simulink model "ACC_ensemble_training"  (R2022a)
settings: Solver=FixedStepAuto  StartTime=0.0  StopTime=T  FixedStep=Ts  RelTol=1e-3
InitFcn:
  | a_lead_seed = randi(10000);
StartFcn:
  | a_lead_seed = randi(10000);
undefined symbols (not defined in the file): actionUB, amax_ego, amax_lead, amin_ego, amin_lead, change_freq, D_default, ensembleRewardWeights, isEnsembleTerminate, isTerminate, MPC_ST, numController, numRL, rewardToIndex, rewardUB1, rewardUB2, rewardWeights, t_gap, tranTable, Ts, v0_ego, v0_lead, v_set, x0_ego, x0_lead
libraries: simulink x10, rllib x10, mpcadaslib x2
settings Model: Creator=The MathWorks, Inc.  LastModifiedBy=momentumlab
settings SolverCC: AlgebraicLoopSolver=TrustRegion
settings DataIOCC: ReturnWorkspaceOutputs=off
settings DebuggingCC: UnconnectedInputMsg=warning  UnconnectedOutputMsg=warning  UnconnectedLineMsg=warning  SFMachineParentedDataDiag=warning  ArithmeticOperatorsInVariantConditions=warning
settings SFSimCC: SimUseLocalCustomCode=off  CustomCodeUndefinedFunction=UseInterfaceOnly
settings RTWCC: RTWUseLocalCustomCode=off  DLArmComputeVersion=19.05
settings CodeAppCC: StateflowObjectComments=on

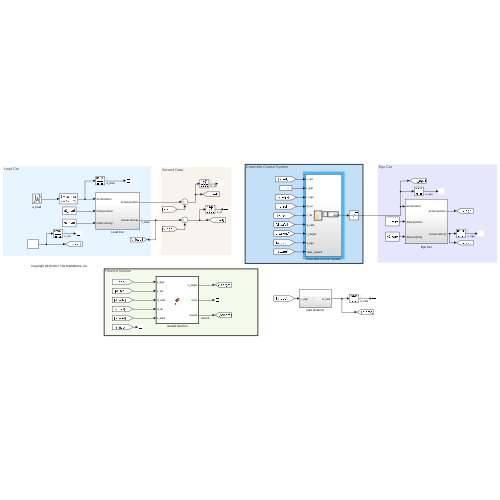
[thumbnail: Simulink's stored preview of the top-level diagram]
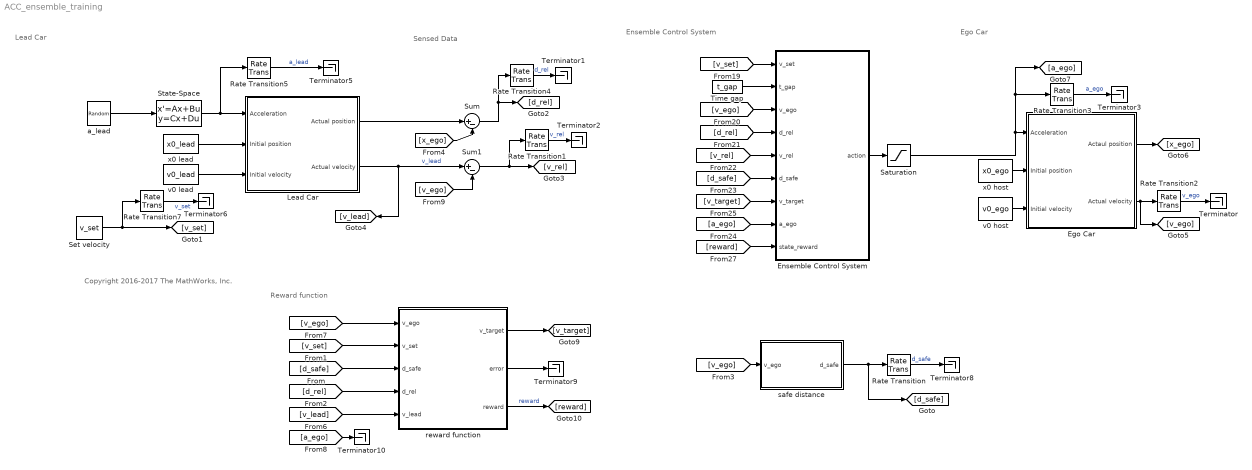
== system ACC_ensemble_training ==
  note: Ensemble Control System
  note: Sensed Data
  note: Lead Car
  note: Ego Car
  note: Copyright 2016-2017 The MathWorks, Inc.
  note: Reward function
  Ego Car : Subsystem
  Ensemble Control System : Subsystem
  Lead Car : Subsystem
  Rate Transition{,1..5,7} (7 alike) : RateTransition  OutPortSampleTime=Ts_data
  Saturation : Saturate  UpperLimit=amax_ego  LowerLimit=amin_ego
  Set velocity : Constant  Value=v_set  SampleTime=Ts
  State-Space : StateSpace  A=-10  B=10  D=0  InitialCondition=0
  Sum : Sum  Inputs=|+-
  Sum1 : Sum  Inputs=|+-
  Terminator{,1..3,5..6,8..10} (9 alike) : Terminator
  Time gap : Constant  Value=t_gap  SampleTime=Ts
  a_lead : UniformRandomNumber  Minimum=amin_lead  Maximum=amax_lead  Seed=a_lead_seed  SampleTime=change_freq  VectorParams1D=off
  reward function : MATLAB Function  TreatAsAtomicUnit=on
  safe distance : Subsystem
  v0 host : Constant  Value=v0_ego  SampleTime=Ts
  v0 lead : Constant  Value=v0_lead  SampleTime=Ts
  x0 host : Constant  Value=x0_ego  SampleTime=Ts
  x0 lead : Constant  Value=x0_lead  SampleTime=Ts
  wires:
  x0 lead/1 -> Lead Car/2(Initial position)
  v0 lead/1 -> Lead Car/3(Initial velocity)
  x0 host/1 -> Ego Car/2(Initial position)
  Ego Car/2(Actual velocity) -> [v_ego], Rate Transition2/1
  v0 host/1 -> Ego Car/3(Initial velocity)
  Set velocity/1 -> Rate Transition7/1, [v_set]
  Saturation/1 -> Ego Car/1(Acceleration), [a_ego], Rate Transition3/1
  Lead Car/1(Actual position) -> Sum/1
  Sum1/1 -> [v_rel], Rate Transition1/1
  State-Space/1 -> Rate Transition5/1, Lead Car/1(Acceleration)
  Lead Car/2(Actual velocity) -> Sum1/1, [v_lead]  "v_lead"
  Sum/1 -> [d_rel], Rate Transition4/1
  a_lead/1 -> State-Space/1
  safe distance/1(d_safe) -> [d_safe], Rate Transition/1
  Rate Transition/1 -> Terminator8/1  "d_safe"
  Rate Transition2/1 -> Terminator/1  "v_ego"
  Rate Transition3/1 -> Terminator3/1  "a_ego"
  Rate Transition5/1 -> Terminator5/1  "a_lead"
  [v_ego] -> safe distance/1(v_ego)
  Ego Car/1(Actaul position) -> [x_ego]
  Rate Transition4/1 -> Terminator1/1  "d_rel"
  Rate Transition1/1 -> Terminator2/1  "v_rel"
  [x_ego] -> Sum/2
  [v_ego] -> Sum1/2
  Rate Transition7/1 -> Terminator6/1  "v_set"
  Ensemble Control System/1(action) -> Saturation/1
  [v_set] -> Ensemble Control System/1(v_set)
  Time gap/1 -> Ensemble Control System/2(t_gap)
  [v_ego] -> Ensemble Control System/3(v_ego)
  [d_rel] -> Ensemble Control System/4(d_rel)
  [v_rel] -> Ensemble Control System/5(v_rel)
  [d_safe] -> Ensemble Control System/6(d_safe)
  [a_ego] -> Ensemble Control System/8(a_ego)
  [v_target] -> Ensemble Control System/7(v_target)
  [reward] -> Ensemble Control System/9(state_reward)
  [d_safe] -> reward function/3(d_safe)
  [v_set] -> reward function/2(v_set)
  reward function/1(v_target) -> [v_target]
  reward function/3(reward) -> [reward]  "reward"
  [v_lead] -> reward function/5(v_lead)
  reward function/2(error) -> Terminator9/1
  [v_ego] -> reward function/1(v_ego)
  [a_ego] -> Terminator10/1
  [d_rel] -> reward function/4(d_rel)

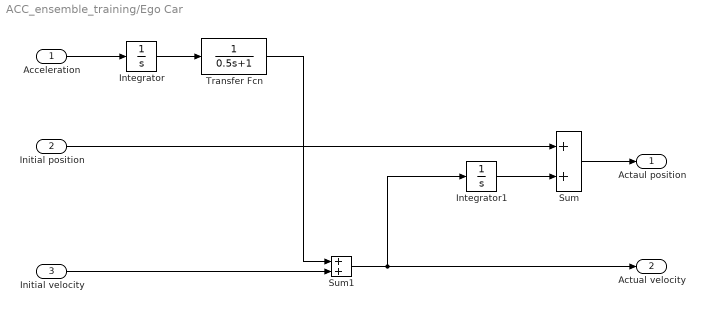
== system ACC_ensemble_training/Ego Car ==
  Acceleration : Inport
  Initial position : Inport  Port=2
  Initial velocity : Inport  Port=3
  Integrator : Integrator
  Integrator1 : Integrator
  Sum : Sum
  Sum1 : Sum
  Transfer Fcn : TransferFcn  Denominator=[0.5 1]
  Actaul position : Outport  VectorParamsAs1DForOutWhenUnconnected=off
  Actual velocity : Outport  Port=2  VectorParamsAs1DForOutWhenUnconnected=off
  wires:
  Sum1/1 -> Integrator1/1, Actual velocity/1
  Initial velocity/1 -> Sum1/2
  Sum/1 -> Actaul position/1
  Transfer Fcn/1 -> Sum1/1
  Integrator/1 -> Transfer Fcn/1
  Acceleration/1 -> Integrator/1
  Initial position/1 -> Sum/1
  Integrator1/1 -> Sum/2

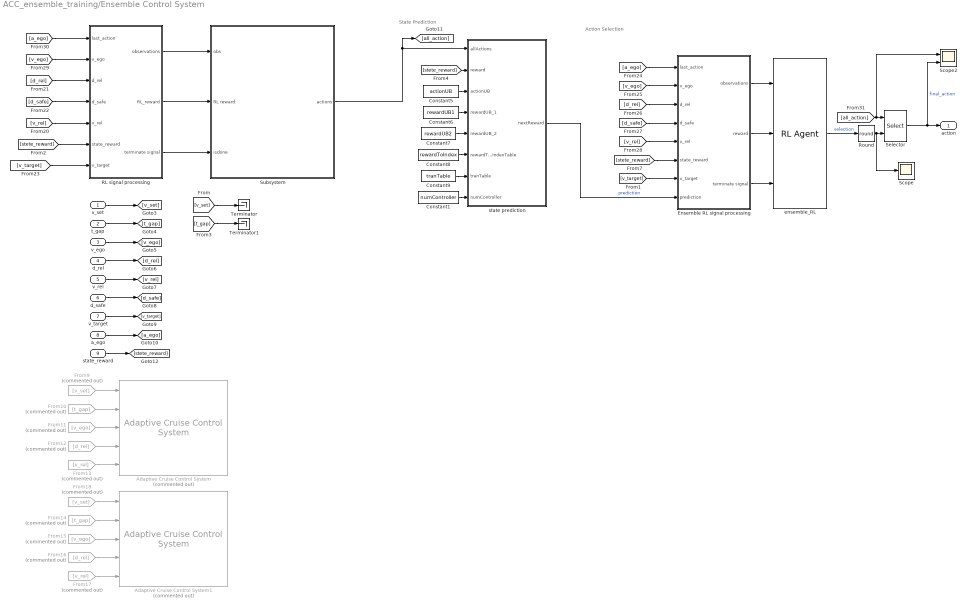
== system ACC_ensemble_training/Ensemble Control System ==
  note: Action Selection
  note: State Prediction
  v_set : Inport
  t_gap : Inport  Port=2
  v_ego : Inport  Port=3
  d_rel : Inport  Port=4
  v_rel : Inport  Port=5
  d_safe : Inport  Port=6
  v_target : Inport  Port=7
  a_ego : Inport  Port=8
  state_reward : Inport  Port=9
  Adaptive Cruise Control System : mpcadaslib/Adaptive Cruise Control System  Commented=on  EgoModel=tf(1,[0.5,1,0])  InitialEgoVelocity=v0_ego  DefaultSpacing=D_default  MaxVelocity=50  MinAcceleration=amin_ego  amin_ext=off  MaxAcceleration=amax_ego  amax_ext=off  Ts=MPC_ST  PredictionHorizon=MPC_PH_1  ControllerBehavior=MPC_behavior_1  suboptimal=off  maxiter=10  datatypeopt=double  optmode=off  trackmode=off
  Adaptive Cruise Control System1 : mpcadaslib/Adaptive Cruise Control System  Commented=on  EgoModel=tf(1,[0.5,1,0])  InitialEgoVelocity=v0_ego  DefaultSpacing=D_default  MaxVelocity=50  MinAcceleration=amin_ego  amin_ext=off  MaxAcceleration=amax_ego  amax_ext=off  Ts=MPC_ST  PredictionHorizon=MPC_PH_2  ControllerBehavior=MPC_behavior_2  suboptimal=off  maxiter=10  datatypeopt=double  optmode=off  trackmode=off
  Constant1 : Constant  Value=numController
  Constant5 : Constant  Value=actionUB
  Constant6 : Constant  Value=rewardUB1
  Constant7 : Constant  Value=rewardUB2
  Constant8 : Constant  Value=rewardToIndex
  Constant9 : Constant  Value=tranTable
  Ensemble RL signal processing : Subsystem
  From10 : From  Commented=on  GotoTag=t_gap
  From11 : From  Commented=on  GotoTag=v_ego
  From12 : From  Commented=on  GotoTag=d_rel
  From13 : From  Commented=on  GotoTag=v_rel
  From14 : From  Commented=on  GotoTag=t_gap
  From15 : From  Commented=on  GotoTag=v_ego
  From16 : From  Commented=on  GotoTag=d_rel
  From17 : From  Commented=on  GotoTag=v_rel
  From18 : From  Commented=on  GotoTag=v_set
  From9 : From  Commented=on  GotoTag=v_set
  "RL signal processing " : Subsystem
  Round : Rounding  Operator=round
  Scope : Scope
  Scope2 : Scope  NumInputPorts=2
  Selector : Selector  IndexOptions=Index vector (port)  Indices=[1 3]  OutputSizes=1
  Subsystem : Subsystem
  Terminator : Terminator
  Terminator1 : Terminator
  ensemble_RL : rllib/RL Agent  Agent=agentEnsemble  ExternalActionAsInput=off  ProvideLastAction=off  ProvideCumRwd=off  TreatAsDirectFeedthrough=on  UseStrictObservationDataTypes=off
  state prediction : MATLAB Function  TreatAsAtomicUnit=on
  action : Outport
  wires:
  v_set/1 -> [v_set]
  t_gap/1 -> [t_gap]
  v_ego/1 -> [v_ego]
  d_rel/1 -> [d_rel]
  v_rel/1 -> [v_rel]
  From9/1 -> Adaptive Cruise Control System/1
  From10/1 -> Adaptive Cruise Control System/2
  From11/1 -> Adaptive Cruise Control System/3
  From12/1 -> Adaptive Cruise Control System/4
  From13/1 -> Adaptive Cruise Control System/5
  From15/1 -> Adaptive Cruise Control System1/3
  From14/1 -> Adaptive Cruise Control System1/2
  From16/1 -> Adaptive Cruise Control System1/4
  From18/1 -> Adaptive Cruise Control System1/1
  From17/1 -> Adaptive Cruise Control System1/5
  d_safe/1 -> [d_safe]
  v_target/1 -> [v_target]
  a_ego/1 -> [a_ego]
  Ensemble RL signal processing/1(observations) -> ensemble_RL/1
  Ensemble RL signal processing/2(reward) -> ensemble_RL/2
  Ensemble RL signal processing/3(terminate signal) -> ensemble_RL/3
  [a_ego] -> Ensemble RL signal processing/1(last_action)
  [v_ego] -> Ensemble RL signal processing/2(v_ego)
  [d_rel] -> Ensemble RL signal processing/3(d_rel)
  [d_safe] -> Ensemble RL signal processing/4(d_safe)
  [v_rel] -> Ensemble RL signal processing/5(v_rel)
  ensemble_RL/1 -> Round/1  "selection"
  Selector/1 -> Scope2/2, action/1  "final_action"
  [all_action] -> Scope2/1, Selector/1
  [v_target] -> Ensemble RL signal processing/7(v_target)
  state_reward/1 -> [stete_reward]
  [stete_reward] -> Ensemble RL signal processing/6(state_reward)
  [stete_reward] -> "RL signal processing "/6(state_reward)
  [v_rel] -> "RL signal processing "/5(v_rel)
  [d_rel] -> "RL signal processing "/3(d_rel)
  [d_safe] -> "RL signal processing "/4(d_safe)
  [v_target] -> "RL signal processing "/7(v_target)
  [v_ego] -> "RL signal processing "/2(v_ego)
  [a_ego] -> "RL signal processing "/1(last_action)
  [stete_reward] -> state prediction/2(reward)
  Constant5/1 -> state prediction/3(actionUB)
  Constant6/1 -> state prediction/4(rewardUB_1)
  Constant7/1 -> state prediction/5(rewardUB_2)
  Constant8/1 -> state prediction/6(rewardToIndexTable)
  Constant9/1 -> state prediction/7(tranTable)
  Constant1/1 -> state prediction/8(numController)
  Round/1 -> Scope/1, Selector/2
  Subsystem/1(actions) -> [all_action], state prediction/1(allActions)
  "RL signal processing "/2(RL_reward) -> Subsystem/2(RL reward)
  "RL signal processing "/3(terminate signal) -> Subsystem/3(isdone)
  "RL signal processing "/1(observations) -> Subsystem/1(obs)
  state prediction/1(nextReward) -> Ensemble RL signal processing/8(prediction)  "prediction"
  [v_set] -> Terminator/1
  [t_gap] -> Terminator1/1

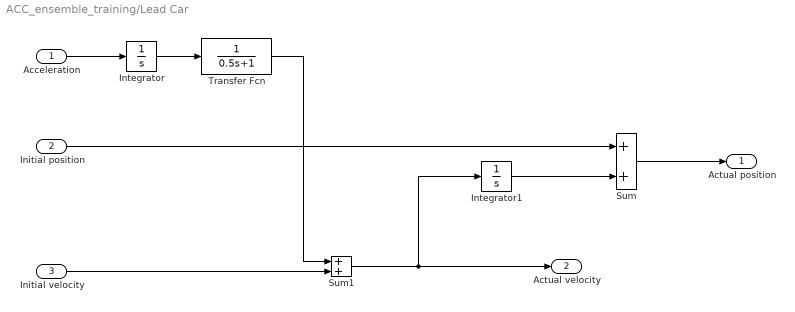
== system ACC_ensemble_training/Lead Car ==
  Acceleration : Inport
  Initial position : Inport  Port=2
  Initial velocity : Inport  Port=3
  Integrator : Integrator
  Integrator1 : Integrator
  Sum : Sum
  Sum1 : Sum
  Transfer Fcn : TransferFcn  Denominator=[0.5 1]
  Actual position : Outport  VectorParamsAs1DForOutWhenUnconnected=off
  Actual velocity : Outport  Port=2  VectorParamsAs1DForOutWhenUnconnected=off
  wires:
  Transfer Fcn/1 -> Sum1/1
  Initial velocity/1 -> Sum1/2
  Sum/1 -> Actual position/1
  Integrator/1 -> Transfer Fcn/1
  Sum1/1 -> Integrator1/1, Actual velocity/1
  Acceleration/1 -> Integrator/1
  Initial position/1 -> Sum/1
  Integrator1/1 -> Sum/2

== system ACC_ensemble_training/safe distance ==
  v_ego : Inport
  Product : Product
  Set velocity1 : Constant  Value=D_default  SampleTime=Ts
  Sum2 : Sum  Inputs=|++
  Time gap : Constant  Value=t_gap  SampleTime=Ts
  d_safe : Outport
  wires:
  Time gap/1 -> Product/1
  Sum2/1 -> d_safe/1
  v_ego/1 -> Product/2
  Product/1 -> Sum2/1
  Set velocity1/1 -> Sum2/2

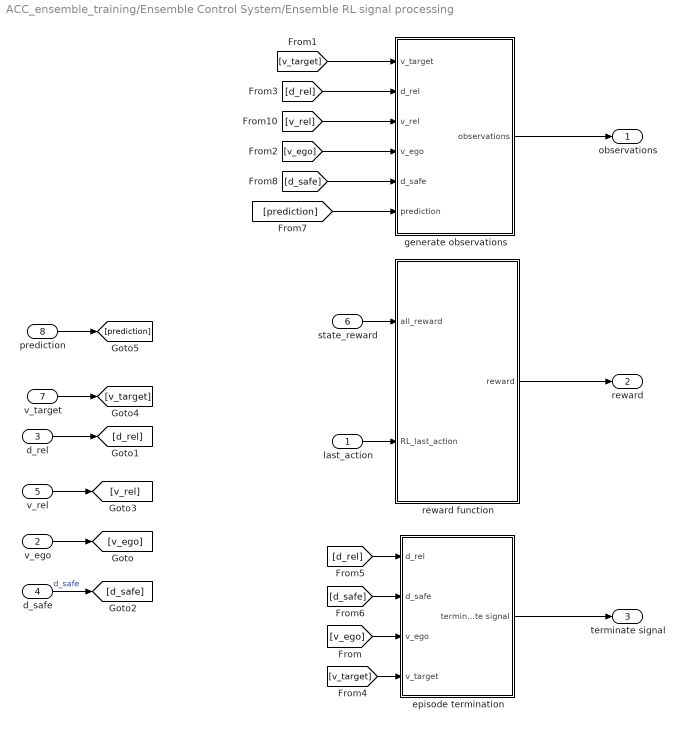
== system ACC_ensemble_training/Ensemble Control System/Ensemble RL signal processing ==
  last_action : Inport
  v_ego : Inport  Port=2
  d_rel : Inport  Port=3
  d_safe : Inport  Port=4
  v_rel : Inport  Port=5
  state_reward : Inport  Port=6
  v_target : Inport  Port=7
  prediction : Inport  Port=8
  episode termination : Subsystem
  generate observations : Subsystem
  reward function : Subsystem
  observations : Outport
  reward : Outport  Port=2
  terminate signal : Outport  Port=3
  wires:
  last_action/1 -> reward function/2(RL_last_action)
  [v_target] -> generate observations/1(v_target)
  v_ego/1 -> [v_ego]
  d_safe/1 -> [d_safe]  "d_safe"
  generate observations/1(observations) -> observations/1
  reward function/1(reward) -> reward/1
  episode termination/1(terminate signal) -> terminate signal/1
  [v_ego] -> episode termination/3(v_ego)
  [v_ego] -> generate observations/4(v_ego)
  [d_rel] -> generate observations/2(d_rel)
  [d_rel] -> episode termination/1(d_rel)
  [d_safe] -> episode termination/2(d_safe)
  [d_safe] -> generate observations/5(d_safe)
  [v_rel] -> generate observations/3(v_rel)
  d_rel/1 -> [d_rel]
  v_rel/1 -> [v_rel]
  state_reward/1 -> reward function/1(all_reward)
  v_target/1 -> [v_target]
  [v_target] -> episode termination/4(v_target)
  prediction/1 -> [prediction]
  [prediction] -> generate observations/6(prediction)

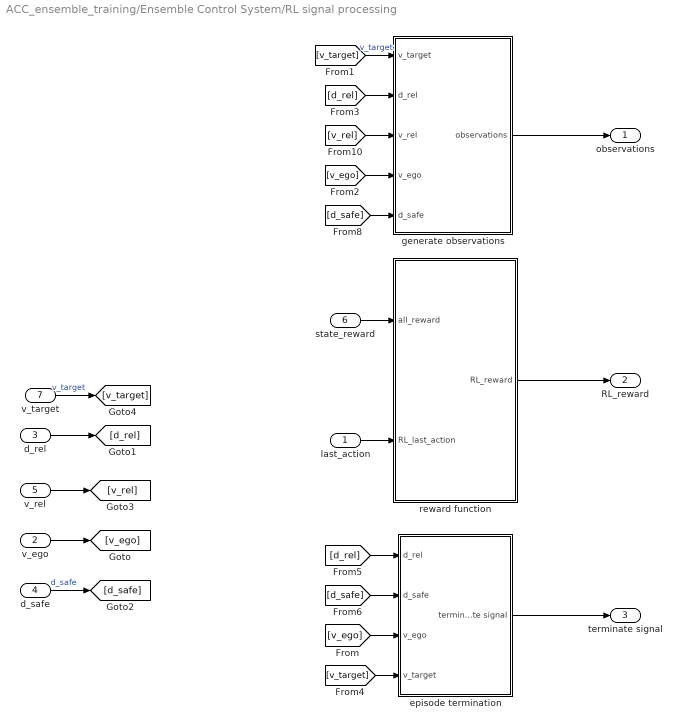
== system ACC_ensemble_training/Ensemble Control System/RL signal processing  ==
  last_action : Inport
  v_ego : Inport  Port=2
  d_rel : Inport  Port=3
  d_safe : Inport  Port=4
  v_rel : Inport  Port=5
  state_reward : Inport  Port=6
  v_target : Inport  Port=7
  episode termination : Subsystem
  generate observations : Subsystem
  reward function : Subsystem
  observations : Outport
  RL_reward : Outport  Port=2
  terminate signal : Outport  Port=3
  wires:
  last_action/1 -> reward function/2(RL_last_action)
  [v_target] -> generate observations/1(v_target)  "v_target"
  v_ego/1 -> [v_ego]
  d_safe/1 -> [d_safe]  "d_safe"
  generate observations/1(observations) -> observations/1
  reward function/1(RL_reward) -> RL_reward/1
  episode termination/1(terminate signal) -> terminate signal/1
  [v_ego] -> episode termination/3(v_ego)
  [v_ego] -> generate observations/4(v_ego)
  [d_rel] -> generate observations/2(d_rel)
  [d_rel] -> episode termination/1(d_rel)
  [d_safe] -> episode termination/2(d_safe)
  [d_safe] -> generate observations/5(d_safe)
  [v_rel] -> generate observations/3(v_rel)
  d_rel/1 -> [d_rel]
  v_rel/1 -> [v_rel]
  state_reward/1 -> reward function/1(all_reward)
  v_target/1 -> [v_target]  "v_target"
  [v_target] -> episode termination/4(v_target)

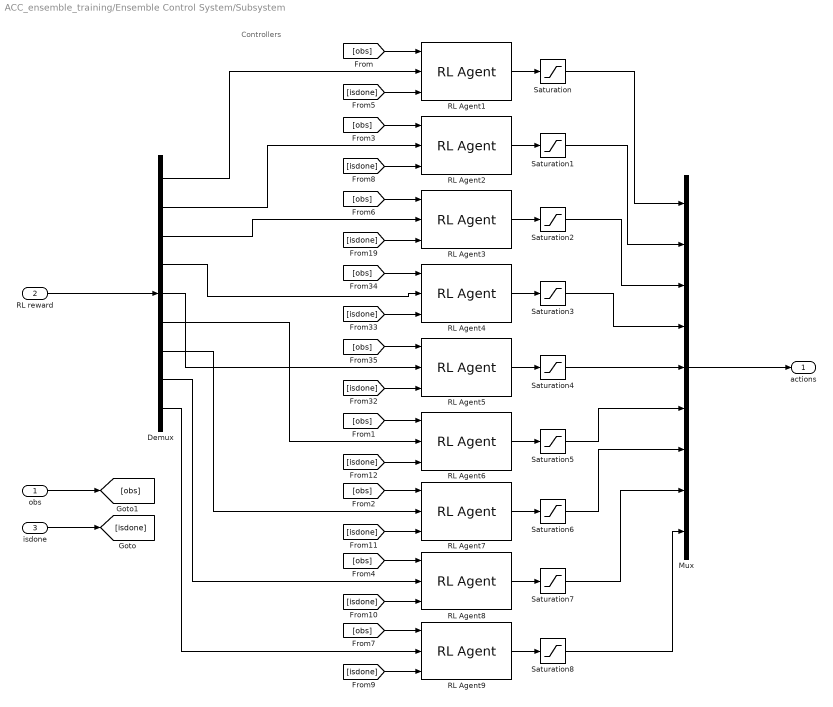
== system ACC_ensemble_training/Ensemble Control System/Subsystem ==
  note: Controllers
  obs : Inport
  RL reward : Inport  Port=2
  isdone : Inport  Port=3
  Demux : Demux  Outputs=9
  Mux : Mux  Inputs=9
  RL Agent1 : rllib/RL Agent  Agent=agent1  ExternalActionAsInput=off  ProvideLastAction=off  ProvideCumRwd=off  TreatAsDirectFeedthrough=on  UseStrictObservationDataTypes=off
  RL Agent2 : rllib/RL Agent  Agent=agent2  ExternalActionAsInput=off  ProvideLastAction=off  ProvideCumRwd=off  TreatAsDirectFeedthrough=on  UseStrictObservationDataTypes=off
  RL Agent3 : rllib/RL Agent  Agent=agent3  ExternalActionAsInput=off  ProvideLastAction=off  ProvideCumRwd=off  TreatAsDirectFeedthrough=on  UseStrictObservationDataTypes=off
  RL Agent4 : rllib/RL Agent  Agent=agent3  ExternalActionAsInput=off  ProvideLastAction=off  ProvideCumRwd=off  TreatAsDirectFeedthrough=on  UseStrictObservationDataTypes=off
  RL Agent5 : rllib/RL Agent  Agent=agent3  ExternalActionAsInput=off  ProvideLastAction=off  ProvideCumRwd=off  TreatAsDirectFeedthrough=on  UseStrictObservationDataTypes=off
  RL Agent6 : rllib/RL Agent  Agent=agent6  ExternalActionAsInput=off  ProvideLastAction=off  ProvideCumRwd=off  TreatAsDirectFeedthrough=on  UseStrictObservationDataTypes=off
  RL Agent7 : rllib/RL Agent  Agent=agent7  ExternalActionAsInput=off  ProvideLastAction=off  ProvideCumRwd=off  TreatAsDirectFeedthrough=on  UseStrictObservationDataTypes=off
  RL Agent8 : rllib/RL Agent  Agent=agent8  ExternalActionAsInput=off  ProvideLastAction=off  ProvideCumRwd=off  TreatAsDirectFeedthrough=on  UseStrictObservationDataTypes=off
  RL Agent9 : rllib/RL Agent  Agent=agent9  ExternalActionAsInput=off  ProvideLastAction=off  ProvideCumRwd=off  TreatAsDirectFeedthrough=on  UseStrictObservationDataTypes=off
  Saturation{,1..8} (9 alike) : Saturate  UpperLimit=amax_ego  LowerLimit=amin_ego
  actions : Outport
  wires:
  [obs] -> RL Agent7/1
  [obs] -> RL Agent4/1
  [obs] -> RL Agent3/1
  Demux/3 -> RL Agent3/2
  Saturation3/1 -> Mux/4
  Demux/5 -> RL Agent5/2
  Demux/1 -> RL Agent1/2
  [obs] -> RL Agent1/1
  [isdone] -> RL Agent1/3
  [obs] -> RL Agent2/1
  [obs] -> RL Agent5/1
  RL Agent1/1 -> Saturation/1
  Demux/2 -> RL Agent2/2
  [isdone] -> RL Agent8/3
  [isdone] -> RL Agent6/3
  RL reward/1 -> Demux/1
  Saturation/1 -> Mux/1
  Demux/8 -> RL Agent8/2
  RL Agent6/1 -> Saturation5/1
  Saturation4/1 -> Mux/5
  RL Agent3/1 -> Saturation2/1
  Demux/6 -> RL Agent6/2
  [isdone] -> RL Agent2/3
  [isdone] -> RL Agent7/3
  RL Agent8/1 -> Saturation7/1
  Saturation1/1 -> Mux/2
  [isdone] -> RL Agent5/3
  Mux/1 -> actions/1
  [obs] -> RL Agent6/1
  Demux/7 -> RL Agent7/2
  [isdone] -> RL Agent3/3
  RL Agent5/1 -> Saturation4/1
  RL Agent4/1 -> Saturation3/1
  RL Agent7/1 -> Saturation6/1
  Demux/4 -> RL Agent4/2
  RL Agent2/1 -> Saturation1/1
  [obs] -> RL Agent8/1
  Saturation2/1 -> Mux/3
  [isdone] -> RL Agent4/3
  Demux/9 -> RL Agent9/2
  RL Agent9/1 -> Saturation8/1
  [obs] -> RL Agent9/1
  [isdone] -> RL Agent9/3
  Saturation5/1 -> Mux/6
  Saturation6/1 -> Mux/7
  Saturation7/1 -> Mux/8
  Saturation8/1 -> Mux/9
  isdone/1 -> [isdone]
  obs/1 -> [obs]

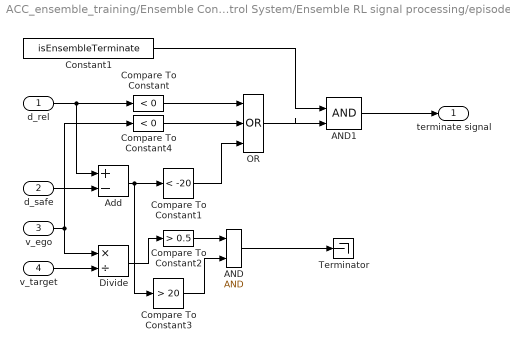
== system ACC_ensemble_training/Ensemble Control System/Ensemble RL signal processing/episode termination ==
  d_rel : Inport
  d_safe : Inport  Port=2
  v_ego : Inport  Port=3
  v_target : Inport  Port=4
  AND : Logic  IconShape=distinctive  AllPortsSameDT=off  OutDataTypeStr=boolean
  AND1 : Logic  IconShape=distinctive  AllPortsSameDT=off  OutDataTypeStr=boolean
  Add : Sum  Inputs=+-
  Compare To Constant : simulink/Logic and Bit Operations/Compare To Constant  relop=<  const=0  OutDataTypeStr=boolean
  Compare To Constant1 : simulink/Logic and Bit Operations/Compare To Constant  relop=<  const=-20  OutDataTypeStr=boolean
  Compare To Constant2 : simulink/Logic and Bit Operations/Compare To Constant  relop=>  const=0.5  OutDataTypeStr=boolean
  Compare To Constant3 : simulink/Logic and Bit Operations/Compare To Constant  relop=>  const=20  OutDataTypeStr=boolean
  Compare To Constant4 : simulink/Logic and Bit Operations/Compare To Constant  relop=<  const=0  OutDataTypeStr=boolean
  Constant1 : Constant  Value=isEnsembleTerminate
  Divide : Product  Inputs=*/
  OR : Logic  Operator=OR  Inputs=3  IconShape=distinctive  AllPortsSameDT=off  OutDataTypeStr=boolean
  Terminator : Terminator
  terminate signal : Outport
  wires:
  d_rel/1 -> Compare To Constant/1, Add/1
  Compare To Constant1/1 -> OR/3
  Add/1 -> Compare To Constant1/1, Compare To Constant3/1
  d_safe/1 -> Add/2
  v_target/1 -> Divide/2
  v_ego/1 -> Compare To Constant4/1, Divide/1
  Divide/1 -> Compare To Constant2/1
  Compare To Constant2/1 -> AND/1
  AND/1 -> Terminator/1
  Compare To Constant3/1 -> AND/2
  Compare To Constant/1 -> OR/1
  Compare To Constant4/1 -> OR/2
  OR/1 -> AND1/2
  AND1/1 -> terminate signal/1
  Constant1/1 -> AND1/1

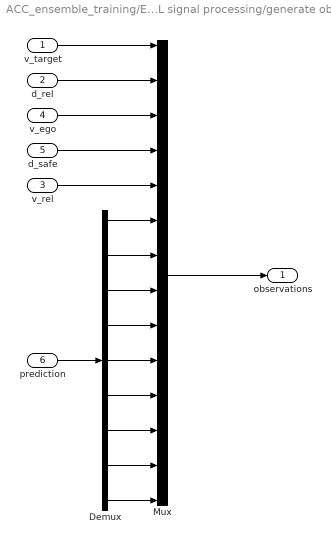
== system ACC_ensemble_training/Ensemble Control System/Ensemble RL signal processing/generate observations ==
  v_target : Inport
  d_rel : Inport  Port=2
  v_rel : Inport  Port=3
  v_ego : Inport  Port=4
  d_safe : Inport  Port=5
  prediction : Inport  Port=6
  Demux : Demux  Outputs=9
  Mux : Mux  Inputs=14
  observations : Outport
  wires:
  v_ego/1 -> Mux/3
  v_target/1 -> Mux/1
  Mux/1 -> observations/1
  d_safe/1 -> Mux/4
  v_rel/1 -> Mux/5
  d_rel/1 -> Mux/2
  prediction/1 -> Demux/1
  Demux/1 -> Mux/6
  Demux/2 -> Mux/7
  Demux/3 -> Mux/8
  Demux/4 -> Mux/9
  Demux/5 -> Mux/10
  Demux/6 -> Mux/11
  Demux/7 -> Mux/12
  Demux/8 -> Mux/13
  Demux/9 -> Mux/14

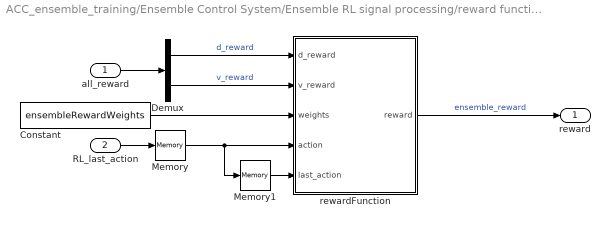
== system ACC_ensemble_training/Ensemble Control System/Ensemble RL signal processing/reward function ==
  all_reward : Inport
  RL_last_action : Inport  Port=2
  Constant : Constant  Value=ensembleRewardWeights
  Demux : Demux  Outputs=2
  Memory : Memory
  Memory1 : Memory
  rewardFunction : MATLAB Function  TreatAsAtomicUnit=on
  reward : Outport
  wires:
  rewardFunction/1(reward) -> reward/1  "ensemble_reward"
  RL_last_action/1 -> Memory/1
  all_reward/1 -> Demux/1
  Demux/1 -> rewardFunction/1(d_reward)  "d_reward"
  Demux/2 -> rewardFunction/2(v_reward)  "v_reward"
  Constant/1 -> rewardFunction/3(weights)
  Memory/1 -> Memory1/1, rewardFunction/4(action)
  Memory1/1 -> rewardFunction/5(last_action)

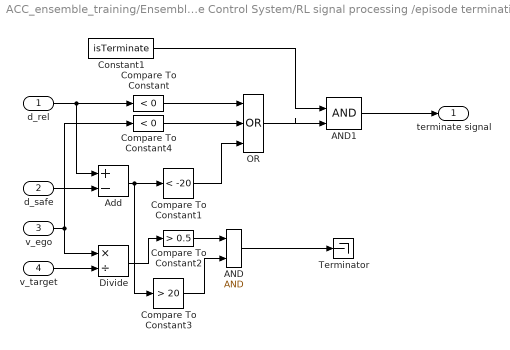
== system ACC_ensemble_training/Ensemble Control System/RL signal processing /episode termination ==
  d_rel : Inport
  d_safe : Inport  Port=2
  v_ego : Inport  Port=3
  v_target : Inport  Port=4
  AND : Logic  IconShape=distinctive  AllPortsSameDT=off  OutDataTypeStr=boolean
  AND1 : Logic  IconShape=distinctive  AllPortsSameDT=off  OutDataTypeStr=boolean
  Add : Sum  Inputs=+-
  Compare To Constant : simulink/Logic and Bit Operations/Compare To Constant  relop=<  const=0  OutDataTypeStr=boolean
  Compare To Constant1 : simulink/Logic and Bit Operations/Compare To Constant  relop=<  const=-20  OutDataTypeStr=boolean
  Compare To Constant2 : simulink/Logic and Bit Operations/Compare To Constant  relop=>  const=0.5  OutDataTypeStr=boolean
  Compare To Constant3 : simulink/Logic and Bit Operations/Compare To Constant  relop=>  const=20  OutDataTypeStr=boolean
  Compare To Constant4 : simulink/Logic and Bit Operations/Compare To Constant  relop=<  const=0  OutDataTypeStr=boolean
  Constant1 : Constant  Value=isTerminate
  Divide : Product  Inputs=*/
  OR : Logic  Operator=OR  Inputs=3  IconShape=distinctive  AllPortsSameDT=off  OutDataTypeStr=boolean
  Terminator : Terminator
  terminate signal : Outport
  wires:
  d_rel/1 -> Compare To Constant/1, Add/1
  Compare To Constant1/1 -> OR/3
  Add/1 -> Compare To Constant1/1, Compare To Constant3/1
  d_safe/1 -> Add/2
  v_target/1 -> Divide/2
  v_ego/1 -> Compare To Constant4/1, Divide/1
  Divide/1 -> Compare To Constant2/1
  Compare To Constant2/1 -> AND/1
  AND/1 -> Terminator/1
  Compare To Constant3/1 -> AND/2
  Compare To Constant/1 -> OR/1
  Compare To Constant4/1 -> OR/2
  OR/1 -> AND1/2
  AND1/1 -> terminate signal/1
  Constant1/1 -> AND1/1

== system ACC_ensemble_training/Ensemble Control System/RL signal processing /generate observations ==
  v_target : Inport
  d_rel : Inport  Port=2
  v_rel : Inport  Port=3
  v_ego : Inport  Port=4
  d_safe : Inport  Port=5
  Mux : Mux  Inputs=5
  observations : Outport
  wires:
  v_ego/1 -> Mux/3
  v_target/1 -> Mux/1
  Mux/1 -> observations/1
  d_safe/1 -> Mux/4
  v_rel/1 -> Mux/5
  d_rel/1 -> Mux/2

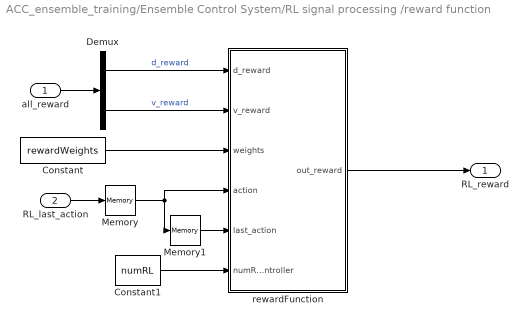
== system ACC_ensemble_training/Ensemble Control System/RL signal processing /reward function ==
  all_reward : Inport
  RL_last_action : Inport  Port=2
  Constant : Constant  Value=rewardWeights
  Constant1 : Constant  Value=numRL
  Demux : Demux  Outputs=2
  Memory : Memory
  Memory1 : Memory
  rewardFunction : MATLAB Function  TreatAsAtomicUnit=on
  RL_reward : Outport
  wires:
  RL_last_action/1 -> Memory/1
  all_reward/1 -> Demux/1
  Demux/1 -> rewardFunction/1(d_reward)  "d_reward"
  Demux/2 -> rewardFunction/2(v_reward)  "v_reward"
  Constant/1 -> rewardFunction/3(weights)
  Memory/1 -> Memory1/1, rewardFunction/4(action)
  Memory1/1 -> rewardFunction/5(last_action)
  Constant1/1 -> rewardFunction/6(numRLController)
  rewardFunction/1(out_reward) -> RL_reward/1

== matlab function ACC_ensemble_training/Ensemble Control System/Ensemble RL signal processing/reward function/rewardFunction ==
  data: d_reward input; reward output; v_reward input; weights input; action input; last_action input
function reward = fcn(d_reward,v_reward,weights, action, last_action)




stable_reward = -2*tanh(abs(action-last_action))+1;

% output reward
% error = [d_error, v_error];
% reward = [d_reward, v_reward];
reward = d_reward*weights(1) + v_reward*weights(2)+stable_reward*weights(3);

== matlab function ACC_ensemble_training/reward function ==
  data: v_target output; error output; v_ego input; reward output; v_set input; d_safe input; d_rel input; v_lead input
function [v_target, error, reward]= fcn(v_ego, v_set, d_safe, d_rel, v_lead)


% If the relative distance is less than the safe distance, 
% the ego car tracks the minimum of the lead car velocity and driver-set velocity
d_safe = d_safe +1;

if d_rel <= d_safe
    v_target = min(v_set, v_lead);
else
    v_target = v_set;
end

v_error = v_ego - v_target;

% reward for velocity [-1,1]
v_reward = -2*tanh(abs(v_error/2)) + 1;

% reward for distance [-1,1]
d_error = d_rel - d_safe;
if d_error >= 0
    d_reward = 1;
else
    d_reward = tanh(d_error/3)-0.5;
end

% output reward
error = [d_error, v_error];
reward = [d_reward, v_reward];

== matlab function ACC_ensemble_training/Ensemble Control System/state prediction ==
  data: nextReward output double; allActions input; reward input; actionUB input; rewardUB_1 input; rewardUB_2 input; rewardToIndexTable input; tranTable input; numController input
function nextReward= fcn(allActions, reward, actionUB, rewardUB_1,rewardUB_2, rewardToIndexTable,tranTable,numController)

% assert(numController == 5);
numController = 9;

nextReward = ones(numController, 1);
abReward_1 = find(rewardUB_1 >= reward(1), 1, 'first');  % concrete state -> abstract state
abReward_2 = find(rewardUB_2 >= reward(2), 1, 'first');
abState = rewardToIndexTable(rewardToIndexTable(:,1)==abReward_1 & rewardToIndexTable(:,2)==abReward_2,3);
stateTable = tranTable(:,1);
actionTable = tranTable(:,2);

for i = 1:numController

    action = allActions(i);
    abAction = find(actionUB >= action, 1, 'first');      % concrete action -> abstract action
    
    temp = (stateTable==abState) + (actionTable==abAction);

    if ismember(2,temp)
        abTranReward = tranTable((stateTable==abState & actionTable==abAction),3);
    else
        abTranReward = 0;
    end
    
    
%     if sum(tranTable(:,1)==abState & tranTable(:,2)==abAction)~=0
%         abTranReward = tranTable(tranTable(:,1)==abState & tranTable(:,2)==abAction,3);
%     else
%         abTranReward = 0;
%     end

%     if isempty(abTranReward)
%         abTranReward = 0;
%     end

    nextReward(i,1) = abTranReward;
end
% p1 = nextReward(1);
% p2 = nextReward(2);
% p3 = nextReward(3);
% p4 = nextReward(4);
% p5 = nextReward(5);

== matlab function ACC_ensemble_training/Ensemble Control System/RL signal processing /reward function/rewardFunction ==
  data: d_reward input; out_reward output double; v_reward input; weights input; action input; last_action input; numRLController input
function out_reward = fcn(d_reward,v_reward,weights, action, last_action,numRLController)

numRLController = 9;

stable_reward = -2*tanh(abs(action-last_action))+1;

out_reward =zeros(numRLController,1);

for i = 1:numRLController
    out_reward(i) = d_reward*weights(i,1) + v_reward*weights(i,2)+stable_reward*weights(i,3);
end

% r1 = out_reward(1,1);
% r2 = out_reward(2,1);
% r3 = out_reward(3,1);
% r4 = out_reward(4,1);
% r5 = out_reward(5,1);
